simulink model "phase_sin_s"  (R2017b)
settings: Solver=VariableStepAuto  StartTime=0.0  StopTime=20  MaxStep=0.001  RelTol=1e-3
values from neighbouring files (symbols this model uses):
  k = 2    [phase.m]    (also in phase_sin.m)
  T = 1    [phase.m]    (also in phase_sin.m)
  w_s = [3/4 7 1/4]    [phase.m]
undefined symbols (not defined in the file or in its folder): n, phi_r
settings Model: Creator=Witaj Przemku  LastModifiedBy=lev
settings CodeAppCC: StateflowObjectComments=on

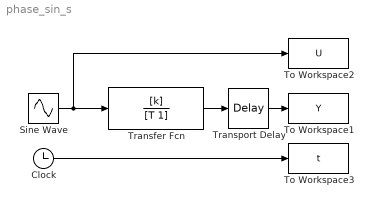
== system phase_sin_s ==
  Clock : Clock
  Sine Wave : Sin  Frequency=w_s(n)  SampleTime=0
  To Workspace1 : ToWorkspace  VariableName=Y  SampleTime=-1
      settings: Save2DSignal=2-D array (concatenate along first dimension)
  To Workspace2 : ToWorkspace  VariableName=U  SampleTime=-1
      settings: Save2DSignal=2-D array (concatenate along first dimension)
  To Workspace3 : ToWorkspace  VariableName=t  SampleTime=-1
      settings: Save2DSignal=2-D array (concatenate along first dimension)
  Transfer Fcn : TransferFcn  Numerator=[k]  Denominator=[T 1]
  Transport Delay : TransportDelay  DelayTime=phi_r(n)  BufferSize=2048
  wires:
  Sine Wave/1 -> Transfer Fcn/1, To Workspace2/1
  Clock/1 -> To Workspace3/1
  Transfer Fcn/1 -> Transport Delay/1
  Transport Delay/1 -> To Workspace1/1
